simulink model "Complete_dynamic"  (R2018b)
settings: Solver=VariableStepAuto  StartTime=0.0  StopTime=50  RelTol=1e-3
undefined symbols (not defined in the file): alpha, CL, Cm, d, g, Iyy, l, l1, m, V
libraries: vrlib x5, simulink_extras x2
settings Model: Creator=ferra  LastModifiedBy=ferra

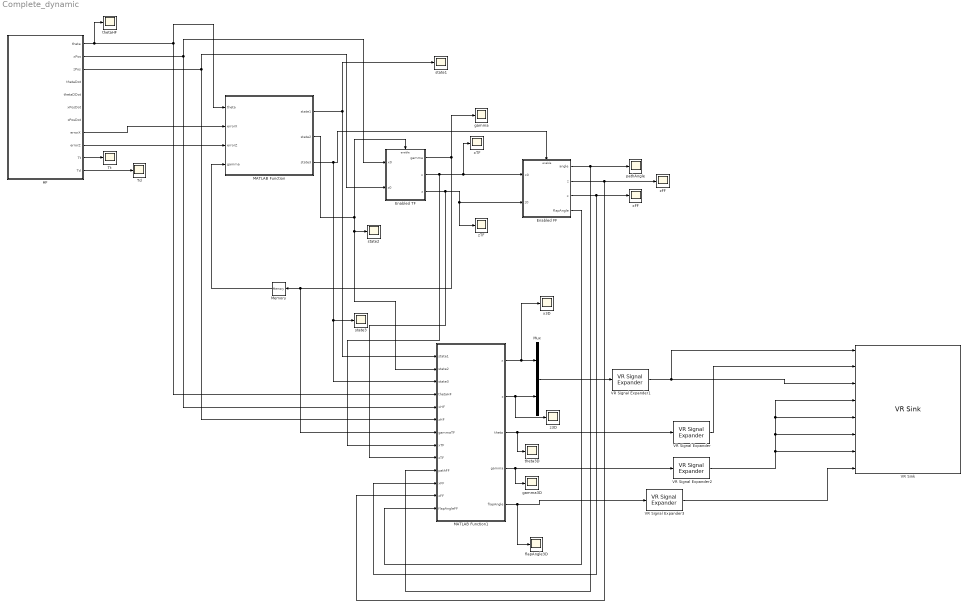
== system Complete_dynamic ==
  Enabled FF : Subsystem  TreatAsAtomicUnit=on
  Enabled TF : Subsystem  TreatAsAtomicUnit=on
  HF : Subsystem
  MATLAB Function : MATLAB Function  TreatAsAtomicUnit=on
  MATLAB Function1 : MATLAB Function  TreatAsAtomicUnit=on
  Memory : Memory
  Mux : Mux  Inputs=2
  Td : Scope
  Tt : Scope
  VR Signal Expander : vrlib/VR Signal Expander  outwidth=4  outidx=[4]
      settings: SourceProductName=Simulink 3D Animation  SourceProductBaseCode=VR
  VR Signal Expander1 : vrlib/VR Signal Expander  outwidth=3  outidx=[1,2]
      settings: SourceProductName=Simulink 3D Animation  SourceProductBaseCode=VR
  VR Signal Expander2 : vrlib/VR Signal Expander  outwidth=4  outidx=[4]
      settings: SourceProductName=Simulink 3D Animation  SourceProductBaseCode=VR
  VR Signal Expander3 : vrlib/VR Signal Expander  outwidth=4  outidx=[4]
      settings: SourceProductName=Simulink 3D Animation  SourceProductBaseCode=VR
  VR Sink : vrlib/VR Sink  InstantiateOnLoad=on  SampleTime=0.05  ViewEnable=on  RemoteChange=off  RemoteView=off  FieldsWritten=FarAway_Front.position.3.1.1.double#Airplane.rotation.4.1.1.double#Airplane.translation.3.1.1.double#Rotor_1.rotation.4.1.1.double#Rotor_2.rotation.4.1.1.double#Rotor_3.rotation.4.1.1.double#Rotor_4.rotation.4.1.1.double#Flap_tail.rotation.4.1.1.double  WorldFileName=C:\Users\ferra\Desktop\Projects\Matlab\Thesis\3D-simulation\3D_world.WRL  AutoView=off  VideoDimensions=[]  AllowVariableSize=off  FigureProperties="{'Position', 'Name', 'Viewpoint', 'CameraBound', 'CameraDirection', 'CameraPosition', 'CameraUpVector', 'ZoomFactor', 'Antialiasing', 'Headlight', 'Lighting', 'NavPanel', 'Sound', 'StatusBar', 'Stereo3D', 'Stereo3DCameraOffset', 'Stereo3DHIT', 'ToolBar', 'Textures', 'Transparency', 'Triad', 'Wireframe', 'NavZones', 'NavMode', 'NavSpeed', 'CaptureFileFormat', 'CaptureFileName', 'Record2DCompressMethod', 'Record2DCompressQuality', 'Record2D', 'Record2DFileName', 'Record2DFPS'; [1.0000000000000000e+00   7.6000000000000000e+01   1.9200000000000000e+03   9.5300000000000000e+02], '', 'far away front POV', 'on', [0.0000000000000000e+00   0.0000000000000000e+00  -1.0000000000000000e+00], [0.0000000000000000e+00   0.0000000000000000e+00  -1.8000000000000000e+01], [0.0000000000000000e+00   1.0000000000000000e+00   0.0000000000000000e+00], [1.0000000000000000e+00], 'on', 'on', 'on', 'halfbar', 'on', 'on', 'off', [1.0000000149011612e-01], [0.0000000000000000e+00], 'on', 'on', 'on', 'none', 'off', 'off', 'walk', 'normal', 'tif', '%f_anim_%n.tif', 'auto', [7.5000000000000000e+01], 'on', 'C:\\Users\\ferra\\Desktop\\Projects\\Matlab\\Thesis\\Recording_simulaiton\\Complete.avi', [6.0000000000000000e+01]}"
      settings: SourceProductBaseCode=VR
  flapAngle3D : Scope
  gamma : Scope
  gamma3D : Scope
  pathAngle : Scope
  state1 : Scope
  state2 : Scope
  state3 : Scope
  theta3D : Scope
  thetaHF : Scope
  x3D : Scope
  xFF : Scope
  xTF : Scope
  z3D : Scope
  zFF : Scope
  zTF : Scope
  wires:
  HF/1(theta) -> thetaHF/1, MATLAB Function/1(theta), MATLAB Function1/4(thetaHF)
  HF/8(errorX) -> MATLAB Function/2(errorX)
  HF/9("errorZ ") -> MATLAB Function/3(errorZ)
  Enabled TF/1(gamma) -> MATLAB Function1/7(gammaTF), Memory/1, gamma/1
  Enabled TF/2(x) -> MATLAB Function1/8(xTF), xTF/1, Enabled FF/1(x0)
  Enabled TF/3(z) -> MATLAB Function1/9(zTF), zTF/1, Enabled FF/2(z0)
  HF/2(xPos) -> Enabled TF/1(x0), MATLAB Function1/5(xHF)
  HF/3(zPos) -> Enabled TF/2(z0), MATLAB Function1/6(zHF)
  MATLAB Function/2(state2) -> MATLAB Function1/2(state2), state2/1, Enabled TF/Enable
  MATLAB Function/3(state3) -> MATLAB Function1/3(state3), state3/1, Enabled FF/Enable
  Enabled FF/2(z) -> MATLAB Function1/12(zFF), zFF/1
  Enabled FF/3(x) -> MATLAB Function1/11(xFF), xFF/1
  Enabled FF/1(angle) -> MATLAB Function1/10(pathFF), pathAngle/1
  MATLAB Function/1(state1) -> state1/1, MATLAB Function1/1(state1)
  Memory/1 -> MATLAB Function/4(gamma)
  Enabled FF/4(flapAngle) -> MATLAB Function1/13(flapAngleFF)
  MATLAB Function1/1(x) -> x3D/1, Mux/1
  MATLAB Function1/2(z) -> z3D/1, Mux/2
  Mux/1 -> VR Signal Expander1/1
  MATLAB Function1/3(theta) -> theta3D/1, VR Signal Expander/1
  MATLAB Function1/4(gamma) -> gamma3D/1, VR Signal Expander2/1
  MATLAB Function1/5(flapAngle) -> flapAngle3D/1, VR Signal Expander3/1
  VR Signal Expander/1 -> VR Sink/2
  VR Signal Expander1/1 -> VR Sink/1, VR Sink/3
  VR Signal Expander2/1 -> VR Sink/7, VR Sink/4, VR Sink/5, VR Sink/6
  VR Signal Expander3/1 -> VR Sink/8
  HF/10(Tt) -> Tt/1
  HF/11(Td) -> Td/1

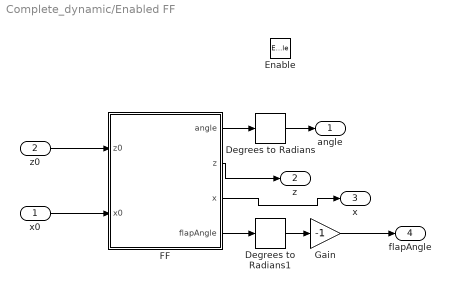
== system Complete_dynamic/Enabled FF ==
  x0 : Inport
  z0 : Inport  Port=2
  Enable : EnablePort  StatesWhenEnabling=reset
  Degrees to Radians : simulink_extras/Transformations/Degrees to Radians
  Degrees to Radians1 : simulink_extras/Transformations/Degrees to Radians
  FF : Subsystem
  Gain : Gain  Gain=-1
  angle : Outport
  z : Outport  Port=2
  x : Outport  Port=3
  flapAngle : Outport  Port=4
  wires:
  FF/1(angle) -> Degrees to Radians/1
  FF/2(z) -> z/1
  FF/3(x) -> x/1
  z0/1 -> FF/1(z0)
  FF/4(flapAngle) -> Degrees to Radians1/1
  x0/1 -> FF/2(x0)
  Degrees to Radians/1 -> angle/1
  Degrees to Radians1/1 -> Gain/1
  Gain/1 -> flapAngle/1

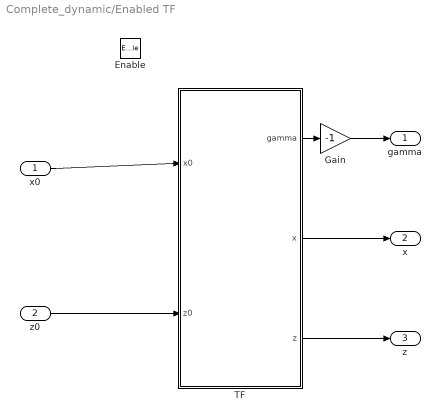
== system Complete_dynamic/Enabled TF ==
  x0 : Inport
  z0 : Inport  Port=2
  Enable : EnablePort  StatesWhenEnabling=reset
  Gain : Gain  Gain=-1
  TF : Subsystem
  gamma : Outport
  x : Outport  Port=2
  z : Outport  Port=3
  wires:
  TF/1(gamma) -> Gain/1
  x0/1 -> TF/1(x0)
  z0/1 -> TF/2(z0)
  TF/2(x) -> x/1
  TF/3(z) -> z/1
  Gain/1 -> gamma/1

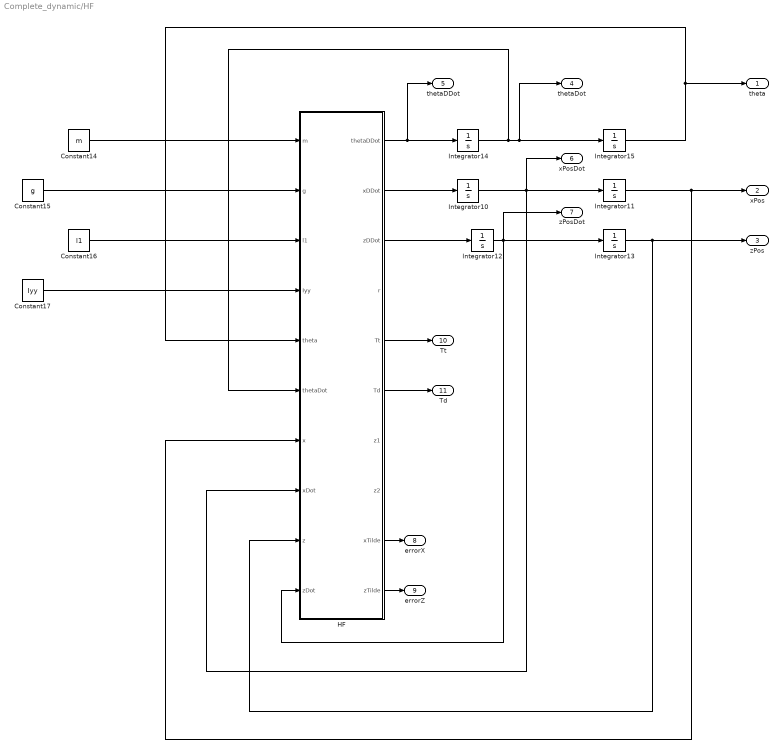
== system Complete_dynamic/HF ==
  Constant14 : Constant  Value=m
  Constant15 : Constant  Value=g
  Constant16 : Constant  Value=l1
  Constant17 : Constant  Value=Iyy
  "HF " : MATLAB Function  TreatAsAtomicUnit=on
  Integrator10 : Integrator
  Integrator11 : Integrator  InitialCondition=-59
  Integrator12 : Integrator
  Integrator13 : Integrator  InitialCondition=1
  Integrator14 : Integrator
  Integrator15 : Integrator  InitialCondition=pi/8
  theta : Outport
  xPos : Outport  Port=2
  zPos : Outport  Port=3
  thetaDot : Outport  Port=4
  thetaDDot : Outport  Port=5
  xPosDot : Outport  Port=6
  zPosDot : Outport  Port=7
  errorX : Outport  Port=8
  "errorZ " : Outport  Port=9
  Tt : Outport  Port=10
  Td : Outport  Port=11
  wires:
  Integrator14/1 -> "HF "/6(thetaDot), thetaDot/1, Integrator15/1
  Integrator15/1 -> theta/1, "HF "/5(theta)
  "HF "/10(zTilde) -> "errorZ "/1
  "HF "/6(Td) -> Td/1
  Integrator13/1 -> "HF "/9(z), zPos/1
  "HF "/2(xDDot) -> Integrator10/1
  Constant16/1 -> "HF "/3(l1)
  "HF "/5(Tt) -> Tt/1
  Integrator10/1 -> "HF "/8(xDot), xPosDot/1, Integrator11/1
  Constant15/1 -> "HF "/2(g)
  Constant14/1 -> "HF "/1(m)
  Integrator11/1 -> "HF "/7(x), xPos/1
  Constant17/1 -> "HF "/4(Iyy)
  "HF "/9(xTilde) -> errorX/1
  Integrator12/1 -> zPosDot/1, Integrator13/1, "HF "/10(zDot)
  "HF "/1(thetaDDot) -> thetaDDot/1, Integrator14/1
  "HF "/3(zDDot) -> Integrator12/1

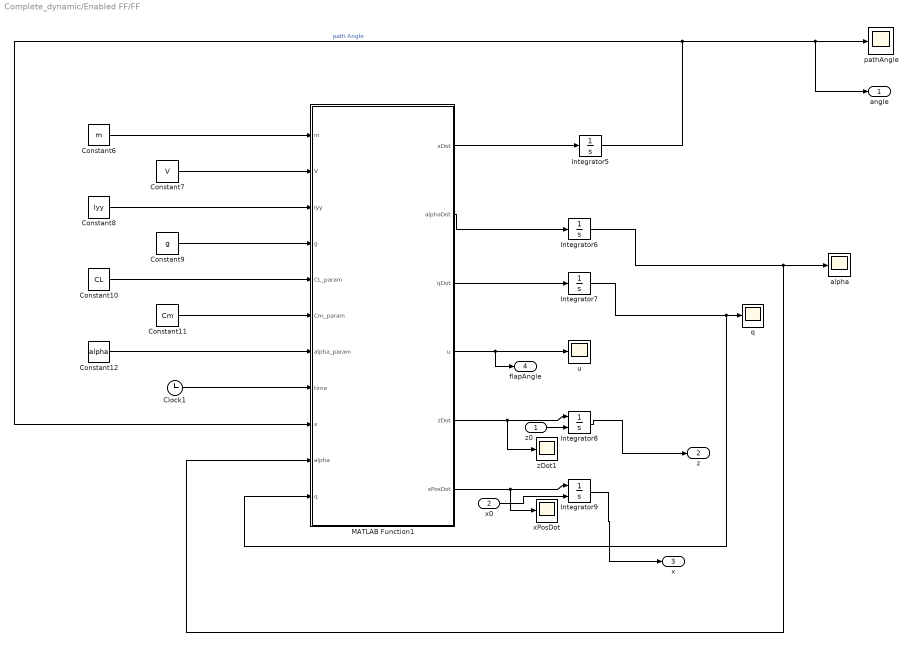
== system Complete_dynamic/Enabled FF/FF ==
  z0 : Inport
  x0 : Inport  Port=2
  Clock1 : Clock
  Constant10 : Constant  Value=CL
  Constant11 : Constant  Value=Cm
  Constant12 : Constant  Value=alpha
  Constant6 : Constant  Value=m
  Constant7 : Constant  Value=V
  Constant8 : Constant  Value=Iyy
  Constant9 : Constant  Value=g
  Integrator5 : Integrator
  Integrator6 : Integrator
  Integrator7 : Integrator
  Integrator8 : Integrator  InitialConditionSource=external  InitialCondition=5
  Integrator9 : Integrator  InitialConditionSource=external  InitialCondition=-30
  MATLAB Function1 : MATLAB Function  TreatAsAtomicUnit=on
  alpha : Scope
  pathAngle : Scope
  q : Scope
  u : Scope
  xPosDot : Scope
  zDot1 : Scope
  angle : Outport
  z : Outport  Port=2
  x : Outport  Port=3
  flapAngle : Outport  Port=4
  wires:
  Constant11/1 -> MATLAB Function1/6(Cm_param)
  Integrator6/1 -> MATLAB Function1/10(alpha), alpha/1
  Constant8/1 -> MATLAB Function1/3(Iyy)
  Integrator7/1 -> MATLAB Function1/11(q), q/1
  Constant7/1 -> MATLAB Function1/2(V)
  Integrator8/1 -> z/1
  Integrator5/1 -> angle/1, pathAngle/1, MATLAB Function1/9(x)  "path Angle"
  MATLAB Function1/2(alphaDot) -> Integrator6/1
  MATLAB Function1/6(xPosDot) -> xPosDot/1, Integrator9/1
  MATLAB Function1/5(zDot) -> zDot1/1, Integrator8/1
  Constant12/1 -> MATLAB Function1/7(alpha_param)
  Constant10/1 -> MATLAB Function1/5(CL_param)
  MATLAB Function1/1(xDot) -> Integrator5/1
  Constant6/1 -> MATLAB Function1/1(m)
  Integrator9/1 -> x/1
  MATLAB Function1/3(qDot) -> Integrator7/1
  Constant9/1 -> MATLAB Function1/4(g)
  MATLAB Function1/4(u) -> flapAngle/1, u/1
  Clock1/1 -> MATLAB Function1/8(time)
  z0/1 -> Integrator8/2
  x0/1 -> Integrator9/2

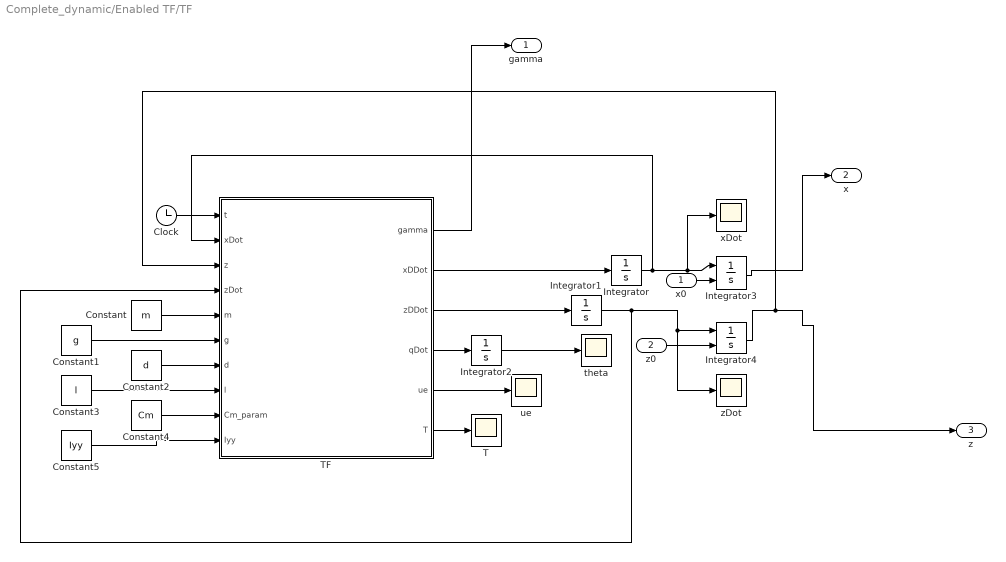
== system Complete_dynamic/Enabled TF/TF ==
  x0 : Inport
  z0 : Inport  Port=2
  Clock : Clock
  Constant : Constant  Value=m
  Constant1 : Constant  Value=g
  Constant2 : Constant  Value=d
  Constant3 : Constant  Value=l
  Constant4 : Constant  Value=Cm
  Constant5 : Constant  Value=Iyy
  Integrator : Integrator
  Integrator1 : Integrator  InitialCondition=1
  Integrator2 : Integrator  InitialCondition=1
  Integrator3 : Integrator  InitialConditionSource=external
  Integrator4 : Integrator  InitialConditionSource=external
  T : Scope
  TF : MATLAB Function  TreatAsAtomicUnit=on
  theta : Scope
  ue : Scope
  xDot : Scope
  zDot : Scope
  gamma : Outport
  x : Outport  Port=2
  z : Outport  Port=3
  wires:
  Constant1/1 -> TF/6(g)
  Integrator1/1 -> TF/4(zDot), zDot/1, Integrator4/1
  Constant/1 -> TF/5(m)
  Integrator/1 -> xDot/1, Integrator3/1, TF/2(xDot)
  TF/4(qDot) -> Integrator2/1
  Clock/1 -> TF/1(t)
  Integrator4/1 -> z/1, TF/3(z)
  Integrator3/1 -> x/1
  TF/2(xDDot) -> Integrator/1
  Constant5/1 -> TF/10(Iyy)
  TF/5(ue) -> ue/1
  Constant3/1 -> TF/8(l)
  Integrator2/1 -> theta/1
  TF/6(T) -> T/1
  TF/3(zDDot) -> Integrator1/1
  Constant4/1 -> TF/9(Cm_param)
  Constant2/1 -> TF/7(d)
  x0/1 -> Integrator3/2
  z0/1 -> Integrator4/2
  TF/1(gamma) -> gamma/1

== matlab function Complete_dynamic/MATLAB Function1 ==
  data: state1 input; x output; state2 input; state3 input; thetaHF input; xHF input; zHF input; gammaTF input; xTF input; zTF input; pathFF input; xFF input; zFF input; z output; theta output; gamma output; flapAngleFF input; flapAngle output
function [x,z,theta,gamma,flapAngle] = fcn(state1,state2,state3,...
                 thetaHF,xHF,zHF,...
                 gammaTF,xTF,zTF,...
                 pathFF,xFF,zFF,flapAngleFF)
    
x = 0;
z = 0;
gamma = 0;
theta = 0;
flapAngle = 0;

rescaleFF = 0.3;
if(state1 ==1)
   x = xHF; 
   z = zHF;
   theta = thetaHF;
   gamma = 0;
   flapAngle = 0;
end
if(state2 == 1)
   x = xTF; 
   z = zTF;
   theta = 0;
   gamma = gammaTF;
   flapAngle = 0;

end
if(state3 == 1)
    x = rescaleFF*xFF;
    z = zFF;
    theta = pathFF;
    gamma = pi/2;
    flapAngle = flapAngleFF;

end

end

== matlab function Complete_dynamic/Enabled FF/FF/MATLAB Function1 ==
  data: m input; xDot output; V input; Iyy input; g input; CL_param input; Cm_param input; alpha_param input; time input; alphaDot output; qDot output; x input; alpha input; q input; u output; zDot output; xPosDot output
function [xDot,alphaDot,qDot,u ,zDot , xPosDot ] = FF(m,V,Iyy,g,CL_param,Cm_param,...
                                    alpha_param, time,x,alpha,q)
Cm = mean(Cm_param);
T = 10;


k1 = 2;
k2 = 2;

if(alpha>71)
    alpha = 71;
elseif(alpha<-10)
    alpha = -10;
end



alphaRound = round(alpha*2)/2;

seqIndex = 1:1:length(alpha_param);
index = round(interp1(alpha_param,seqIndex,alphaRound));
CL = CL_param(index);

f = (-g/V) * cos((CL*x)/(m*V));
f1 = (g/V) * cos((CL*x)/(m*V)) - (CL*alpha)/(m*V);
f2 = 0;
g2 = Cm/Iyy;



df_dx =( (g*CL)/(m*V^2) ) * sin((CL*x)/(m*V));
df1_dx = ((-g*CL)/(m*V^2) ) *sin((CL*x)/(m*V));
df_ddx = ((g*CL^2)/(m*V^3)) * cos((CL * x)/(m*V));

%Definition of the xDes
amp = 1;
freq = 2*pi/10;
% xDes = amp * sin(freq*time);

xDes = 15;

e = x-xDes;

% xDesDot = amp *cos(freq*time);
xDesDot = 0;
alphaDes = -f - k1*e + xDesDot; %Virtual : stabilaize the dynamics of x 
alphaDesDot = (-df_dx -k1)*(f+alpha);


e1 = alpha - alphaDes;
qDes = -f1 -x+xDes - k1*e1 + alphaDesDot; %Virtual: stabilize the dynamics of alpha

e2 = q - qDes;

e1Dot = -e - k1*e1 +e2;





d_alphaDesDot_dx = -df_ddx *f - (df_dx)^2 -df_ddx * alpha - k1*df_dx;
par_qDes_x = -df1_dx - 1 + d_alphaDesDot_dx;
par_qDes_e1 = -k1;
qDesDot = par_qDes_x * (f+alpha) + par_qDes_e1 * (e1Dot);
u = (-f2 + qDesDot - e1 - k2*e2)/(g2);

u = sat(u,25);

xDot = f + alpha;
alphaDot = f1 + q;
qDot = f2 + g2 *u;
zDot  = V * sin(deg2rad(x));
xPosDot = V * cos(deg2rad(x));

end

== matlab function Complete_dynamic/HF/HF  ==
  data: thetaDDot output; m input; xDDot output; g input; l1 input; Iyy input; theta input; thetaDot input; x input; xDot input; z input; zDot input; zDDot output; r output; Tt output; Td output; z1 output; z2 output; xTilde output; zTilde output
function [thetaDDot,xDDot,zDDot, r, Tt,Td , z1,z2,xTilde,zTilde] = HF_dynamics(m,g,l1,Iyy,theta,thetaDot,x,xDot,z,zDot)

zDes = 5;
xDes = -30;

%saturation values
m1 = 0.9;
m2 = 2;
a = 1;
b = 2;
c= 1;

%gain of virutal controllers
kpz = 4;
kdz = 6;


k2 =  1;
k3 = 1;

%function between Td and thetaDot
g2 = -l1/Iyy;

%References
zTilde = z- zDes;
xTilde = x-xDes;


% %Control to stabilize z
r1 = sat(kpz*zTilde,m2) + kdz*zDot;
r = -sat(r1,m1);
Tt = (m*(g-r))/(cos(theta));

% %backstepping
phi1 =  sat(xTilde,a)+ sat(xDot,b);
z1 =phi1 - k2*theta;

% %z1Dot = satDot(x1Tilde,a)*xDot -k2*thetaDot + satDot(xDot,b)*(tan(theta)*(r-g));

% %Virtual Controller
n = -c*z1  - tan(theta)*satDot(xDot,b)*(r-g);
z2 = satDot(xTilde,a)*xDot - k2*thetaDot - n;

z1Dot = z2 - c*z1;

psi = satDot(xTilde,a)*tan(theta)*(r-g) ...
    + sec(theta)*sec(theta)*thetaDot*satDot(xDot,b)*(r-g)...
    +c*(z1Dot)+tan(theta)*satDot(xDot,b)*satDot(zTilde+zDot,m1)*(r-g);

%Controller 
Td = (psi + z1 + k3*z2)/(k2 * g2);

%Dynamics
xDDot = -Tt * sin(theta)/m;
zDDot = -Tt * cos(theta)/m + g;
thetaDDot = Td *g2;



end

== matlab function Complete_dynamic/MATLAB Function ==
  data: theta input; state1 output; errorX input; errorZ input; state2 output; state3 output; gamma input
function [state1,state2,state3] = switchState(theta,errorX,errorZ,gamma)
state1 = 1;
state2 = 0;
state3 = 0;

tolSwitch = 0.05;

if(abs(theta)<tolSwitch && abs(errorX)<tolSwitch && abs(errorZ)<tolSwitch)
    state2 = 1;
   state1 =0';
    
end
if(abs(gamma)>deg2rad(85))
   state2 = 0;
      state1 =0;

   state3 = 1;
end

end

== matlab function Complete_dynamic/Enabled TF/TF/TF ==
  data: t input; gamma output; xDDot output; zDDot output; qDot output; ue output; xDot input; z input; zDot input; m input; g input; d input; l input; T output; Cm_param input; Iyy input
function [gamma,xDDot,zDDot, qDot,ue, T] = TF(t,xDot,z,zDot,m,g,d,l,Cm_param,Iyy)

ue = 0;
zDes = 6;
kpz = 10;
kdz = 4;

k1 = 2;
k2 = 3;


Cm = mean(Cm_param);

T = 0;
%Change angle of thrusts
gamma = (t-32.5)/4;
if(abs(gamma)> pi/2)
   gamma = pi/2; 
end


%virtual controller
vz = kpz*(z-zDes)+kdz*zDot;


phi = -k1*(z-zDes);
e1 = zDot-phi;
phiDot = -k1*(e1 - k1*(z-zDes));


%Check if lift force > mg
if(l*xDot^2-m*g>0)
    %ue = -(T*cos(gamma)+l*xDot^2-m*g+vz)/(xDot^2);

elseif(abs(gamma)< deg2rad(85))
    T = (-z - l*xDot^2+m*g+phiDot-k2*e1)/(cos(gamma));

end


xDDot = T*sin(gamma) - d*xDot^2;
zDDot = T*cos(gamma) + l*xDot^2 + ue*xDot^2 -m*g;


g2 = Cm/Iyy;

qDot =  g2 *ue;


end
